simulink model "HESS"  (R2023a)
settings: Solver=daessc  StartTime=0.0  StopTime=1800  MaxStep=0.1  RelTol=1e-3
values from neighbouring files (symbols this model uses):
  Max_Power = 100000    [setHESSParam.m]    (also in setHESSParamv2.m)
  sim_case = i    [create_SOC_dataset.m]    (also in create_csv.m = 2; setHESSParam.m = 6; setHESSParamv2.m = 6)
undefined symbols (not defined in the file or in its folder): Battery, Capacitor, Ri
libraries: fl_lib x41, nesl_utility x22, rllib x2, dspstat3 x2, batteryecm_lib x1, autolibshared x1
(part 2 of 2)

== matlab function HESS/RL-based EMS/SAC/MATLAB Function ==
  data: Pwr_Dmd input; Bat_Rate input; B_Rate output; Cap_Rate input; Cap_SOC input; C_Rate output; Cap_over_discharge output; Bat_over_discharge output; Cap_over_charge output; Bat_over_charge output; Bat_SOC input
function [B_Rate, C_Rate, Cap_over_discharge, Bat_over_discharge, Cap_over_charge, Bat_over_charge] = filter(Pwr_Dmd, Bat_Rate, Cap_Rate, Cap_SOC, Bat_SOC)

B_Rate = Bat_Rate;
C_Rate = Cap_Rate;

Bat_over_discharge = 0;
Bat_over_charge = 0;

Cap_over_discharge = 0;
Cap_over_charge = 0;

%{
if (Pwr_Dmd >= 0 && Cap_SOC <= 0.5)

    C_Rate = 0;
    Cap_over_discharge = Cap_Rate;

end

if (Pwr_Dmd >= 0 && Bat_SOC <= 0.2)

    B_Rate = 0;
    Bat_over_discharge = Bat_Rate;

end

if (Pwr_Dmd < 0 && Bat_SOC >= 1)

    B_Rate = 0;
    Bat_over_charge = Bat_Rate;

end

if (Pwr_Dmd < 0 && Cap_SOC >= 1)

    C_Rate = 0;
    Cap_over_charge = Cap_Rate;

end
%}
